simulink model "AXIS_To_Stream"  (R2018b)
settings: Solver=VariableStepAuto  StartTime=0.0  StopTime=131000*10*10e-9  RelTol=1e-3
libraries: xbsIndex_r4 x29, hdlsllib x1, simulink_extras x1
settings Model: Creator=marsiau  LastModifiedBy=marsiau

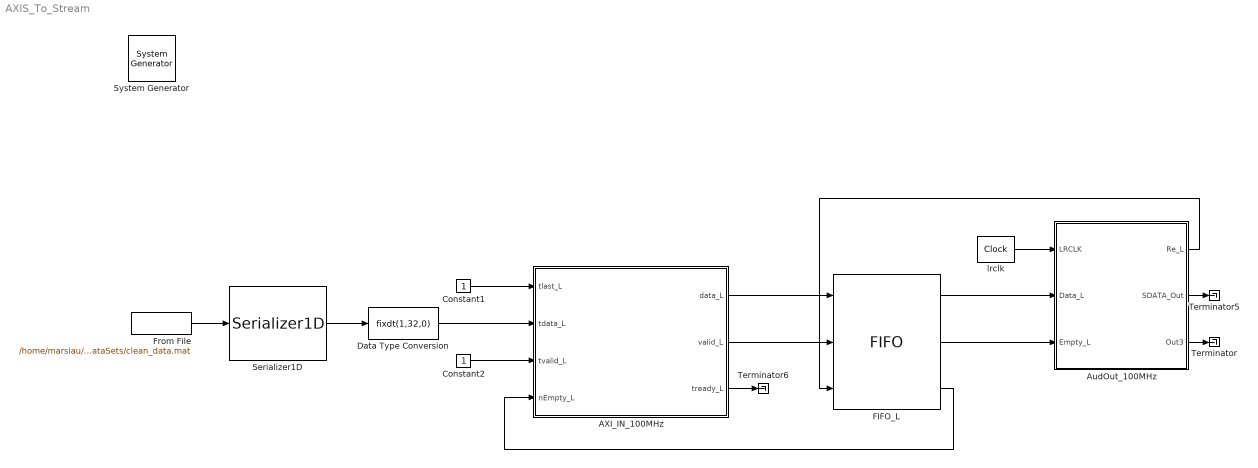
== system AXIS_To_Stream ==
  " System Generator" : xbsIndex_r4/ System Generator  Tag=genX  xilinxfamily=zynq  part=xc7z020  speed=-1  package=clg400  synthesis_tool=Vivado  clock_wrapper=Clock Enables  directory=./netlist  proj_type=Vivado  Synth_file=Vivado Synthesis Defaults  Impl_file=Vivado Implementation Defaults  testbench=off  simulink_period=1  sysclk_period=10  dcm_input_clock_period=10  incr_netlist=off  trim_vbits=Everywhere in SubSystem  dbl_ovrd=According to Block Masks  core_generation=According to Block Masks  run_coregen=off  deprecated_control=off  eval_field=0  block_type=sysgen
  AXI_IN_100MHz : Subsystem
  AudOut_100MHz : Subsystem
  Constant1 : Constant  OutDataTypeStr=boolean  SampleTime=10e-9
  Constant2 : Constant  OutDataTypeStr=boolean  SampleTime=10e-9
  Data Type Conversion : DataTypeConversion  OutDataTypeStr=fixdt(1,32,0)  SaturateOnIntegerOverflow=on  LockScale=on
  FIFO_L : xbsIndex_r4/FIFO  mem_type=Block RAM  performance_options=Standard_FIFO  embedded_registers=off  depth=16K  percent_nbits=1  rst=off  rst_latency=1  en=off  use_dcount=off  use_percent_full_port=off  use_almost_empty=off  almost_empty_thresh=2  use_almost_full=off  use_rd_rst_busy=off  use_wr_rst_busy=off  almost_full_thresh=14  explicit_period=off  dbl_ovrd=off  block_type=fifo
  From File : FromFile  FileName=/home/marsiau/Projects/PYNQ-RTL-SDR/IP/DataSets/clean_data.mat
  Serializer1D : hdlsllib/HDL Operations/Serializer1D  Ratio=131000  IdleCycles=0  validIn=off  startOut=off  validOut=off  inputDataDimensions=-1  inputSampleTime=-1  inputSignalType=auto
      settings: SourceProductName=HDL Coder  SourceProductBaseCode=HD
  Terminator : Terminator
  Terminator5 : Terminator
  Terminator6 : Terminator
  lrclk : simulink_extras/Flip Flops/Clock  period=20.48e-6
  wires:
  FIFO_L/2 -> AudOut_100MHz/3(Empty_L)
  AXI_IN_100MHz/3(tready_L) -> Terminator6/1
  FIFO_L/1 -> AudOut_100MHz/2(Data_L)
  lrclk/1 -> AudOut_100MHz/1(LRCLK)
  AXI_IN_100MHz/2(valid_L) -> FIFO_L/2
  From File/1 -> Serializer1D/1
  AudOut_100MHz/2(SDATA_Out) -> Terminator5/1
  AXI_IN_100MHz/1(data_L) -> FIFO_L/1
  Data Type Conversion/1 -> AXI_IN_100MHz/2(tdata_L)
  FIFO_L/3 -> AXI_IN_100MHz/4(nEmpty_L)
  Constant1/1 -> AXI_IN_100MHz/1(tlast_L)
  AudOut_100MHz/3(Out3) -> Terminator/1
  AudOut_100MHz/1(Re_L) -> FIFO_L/3
  Serializer1D/1 -> Data Type Conversion/1
  Constant2/1 -> AXI_IN_100MHz/3(tvalid_L)

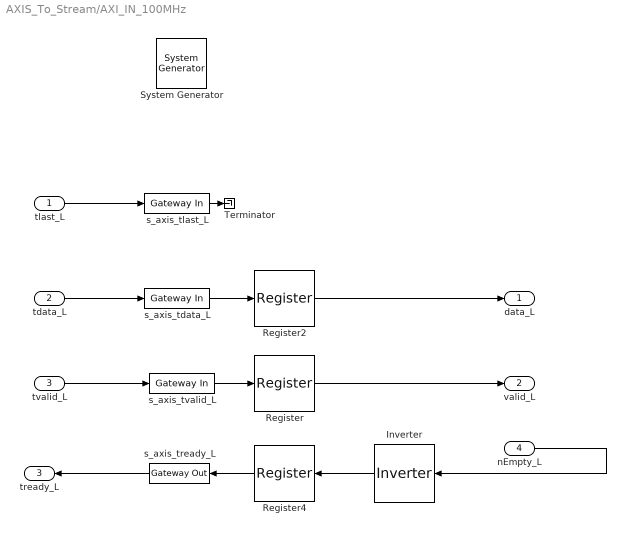
== system AXIS_To_Stream/AXI_IN_100MHz ==
  tlast_L : Inport
  tdata_L : Inport  Port=2
  tvalid_L : Inport  Port=3
  nEmpty_L : Inport  Port=4
  " System Generator" : xbsIndex_r4/ System Generator  Tag=genX  xilinxfamily=zynq  part=xc7z020  speed=-1  package=clg400  synthesis_tool=Vivado  clock_wrapper=Clock Enables  directory=./netlist  proj_type=Vivado  Synth_file=Vivado Synthesis Defaults  Impl_file=Vivado Implementation Defaults  testbench=off  simulink_period=10e-9  sysclk_period=10  dcm_input_clock_period=10  incr_netlist=off  trim_vbits=Everywhere in SubSystem  dbl_ovrd=According to Block Masks  core_generation=According to Block Masks  run_coregen=off  deprecated_control=off  eval_field=0  block_type=sysgen
  Inverter : xbsIndex_r4/Inverter  en=off  latency=0  dbl_ovrd=off  block_type=inv
  Register : xbsIndex_r4/Register  init=0  rst=off  en=off  dbl_ovrd=off  block_type=register
  Register2 : xbsIndex_r4/Register  init=0  rst=off  en=off  dbl_ovrd=off  block_type=register
  Register4 : xbsIndex_r4/Register  init=0  rst=off  en=off  dbl_ovrd=off  block_type=register
  Terminator : Terminator
  s_axis_tdata_L : xbsIndex_r4/Gateway In  gui_display_data_type=Fixed-point  arith_type=Unsigned  n_bits=32  bin_pt=0  preci_type=Single  exp_width=8  frac_width=24  rows=1  columns=1  quantization="Round  (unbiased: +/- Inf)"  overflow=Saturate  period=10e-9  UseAsADC=off  ADCChannel='1'  interface=None  automatic_assignment=on  address_offset=hex2dec('00')  intf_name=''  intf_description=''  default_value=0  timing_constraint=None  locs_specified=off  LOCs={}  io_standard={}  inherit_from_input=off  hdl_port=on  dbl_ovrd=off  block_type=gatewayin
  s_axis_tlast_L : xbsIndex_r4/Gateway In  gui_display_data_type=Boolean  arith_type=Boolean  n_bits=16  bin_pt=14  preci_type=Single  exp_width=8  frac_width=24  rows=1  columns=1  quantization="Round  (unbiased: +/- Inf)"  overflow=Saturate  period=10e-9  UseAsADC=off  ADCChannel='1'  interface=None  automatic_assignment=on  address_offset=hex2dec('00')  intf_name=''  intf_description=''  default_value=0  timing_constraint=None  locs_specified=off  LOCs={}  io_standard={}  inherit_from_input=off  hdl_port=on  dbl_ovrd=off  block_type=gatewayin
  s_axis_tready_L : xbsIndex_r4/Gateway Out  inherit_from_input=off  hdl_port=on  rows=1  columns=1  UseAsDAC=off  DACChannel='1'  interface=None  automatic_assignment=on  address_offset=hex2dec('00')  intf_name=''  intf_description=''  timing_constraint=None  locs_specified=off  LOCs={}  io_standard={}  block_type=gatewayout
  s_axis_tvalid_L : xbsIndex_r4/Gateway In  gui_display_data_type=Boolean  arith_type=Boolean  n_bits=16  bin_pt=14  preci_type=Single  exp_width=8  frac_width=24  rows=1  columns=1  quantization="Round  (unbiased: +/- Inf)"  overflow=Saturate  period=10e-9  UseAsADC=off  ADCChannel='1'  interface=None  automatic_assignment=on  address_offset=hex2dec('00')  intf_name=''  intf_description=''  default_value=0  timing_constraint=None  locs_specified=off  LOCs={}  io_standard={}  inherit_from_input=off  hdl_port=on  dbl_ovrd=off  block_type=gatewayin
  data_L : Outport
  valid_L : Outport  Port=2
  tready_L : Outport  Port=3
  wires:
  s_axis_tvalid_L/1 -> Register/1
  s_axis_tdata_L/1 -> Register2/1
  s_axis_tlast_L/1 -> Terminator/1
  Inverter/1 -> Register4/1
  s_axis_tready_L/1 -> tready_L/1
  tlast_L/1 -> s_axis_tlast_L/1
  tvalid_L/1 -> s_axis_tvalid_L/1
  tdata_L/1 -> s_axis_tdata_L/1
  nEmpty_L/1 -> Inverter/1
  Register/1 -> valid_L/1
  Register4/1 -> s_axis_tready_L/1
  Register2/1 -> data_L/1

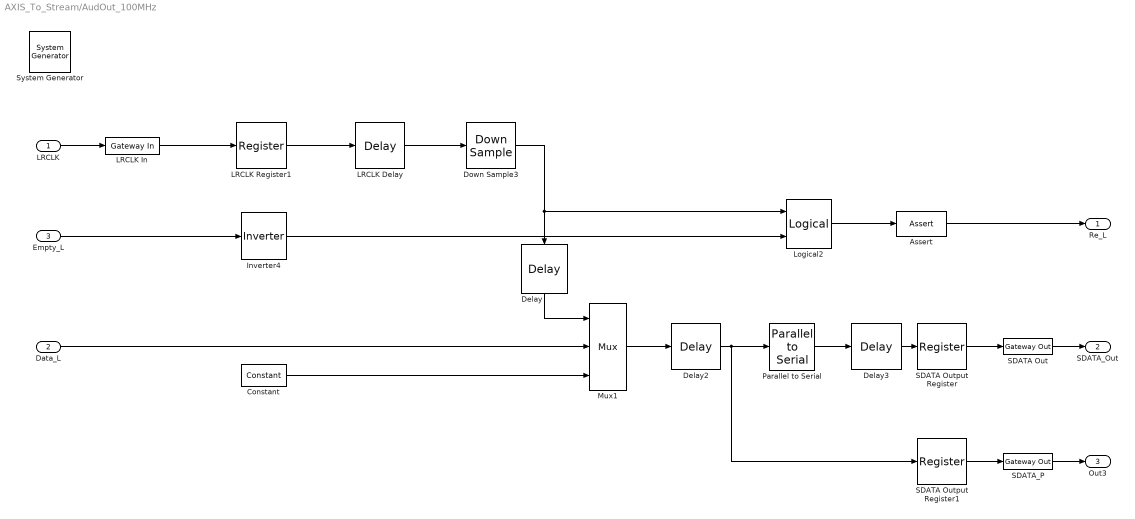
== system AXIS_To_Stream/AudOut_100MHz ==
  LRCLK : Inport
  Data_L : Inport  Port=2
  Empty_L : Inport  Port=3
  " System Generator" : xbsIndex_r4/ System Generator  Tag=genX  xilinxfamily=zynq  part=xc7z020  speed=-1  package=clg400  synthesis_tool=Vivado  clock_wrapper=Clock Enables  directory=./netlist  proj_type=Vivado  Synth_file=Vivado Synthesis Defaults  Impl_file=Vivado Implementation Defaults  testbench=off  simulink_period=10e-9  sysclk_period=10  dcm_input_clock_period=10  incr_netlist=off  trim_vbits=Everywhere in SubSystem  dbl_ovrd=According to Block Masks  core_generation=According to Block Masks  run_coregen=off  deprecated_control=off  eval_field=0  block_type=sysgen
  Assert : xbsIndex_r4/Assert  assert_type=off  type_source=Explicitly  gui_display_data_type=Fixed-point  arith_type="Signed  (2's comp)"  n_bits=16  bin_pt=14  preci_type=Single  exp_width=8  frac_width=24  assert_rate=on  rate_source=Explicitly  period=10.24e-6  output_port=on  block_type=assert
  Constant : xbsIndex_r4/Constant  const=0  gui_display_data_type=Fixed-point  arith_type=Unsigned  n_bits=32  bin_pt=0  preci_type=Single  exp_width=8  frac_width=24  explicit_period=on  period=10.24e-6  equ=P=C  opselect=C  inp2=PCIN>>17  opr=+  inp1=P  carry=CIN  dbl_ovrd=off  block_type=constant
  Delay : xbsIndex_r4/Delay  rst=off  infoeditControl=Selection of Reset will increase slice count due to use of real FFs and instead of SRLs  en=off  latency=1  reg_retiming=off  dbl_ovrd=off  block_type=delay
  Delay2 : xbsIndex_r4/Delay  rst=off  infoeditControl=Selection of Reset will increase slice count due to use of real FFs and instead of SRLs  en=off  latency=1  reg_retiming=off  dbl_ovrd=off  block_type=delay
  Delay3 : xbsIndex_r4/Delay  rst=off  infoeditControl=Selection of Reset will increase slice count due to use of real FFs and instead of SRLs  en=off  latency=32  reg_retiming=off  dbl_ovrd=off  block_type=delay
  Down Sample3 : xbsIndex_r4/Down Sample  sample_ratio=1024  sample_phase=First Value of Frame  en=off  rst=off  latency=0  dbl_ovrd=off  block_type=dsamp
  Inverter4 : xbsIndex_r4/Inverter  en=off  latency=1  dbl_ovrd=off  block_type=inv
  LRCLK Delay : xbsIndex_r4/Delay  rst=off  infoeditControl=Selection of Reset will increase slice count due to use of real FFs and instead of SRLs  en=off  latency=31  reg_retiming=off  dbl_ovrd=off  block_type=delay
  LRCLK In : xbsIndex_r4/Gateway In  gui_display_data_type=Boolean  arith_type=Boolean  n_bits=1  bin_pt=0  preci_type=Single  exp_width=8  frac_width=24  rows=1  columns=1  quantization=Truncate  overflow=Saturate  period=10e-9  UseAsADC=off  ADCChannel='1'  interface=None  automatic_assignment=off  address_offset=hex2dec('04')  intf_name=''  intf_description=''  default_value=0  timing_constraint=None  locs_specified=off  LOCs={}  io_standard={}  inherit_from_input=off  hdl_port=on  dbl_ovrd=off  block_type=gatewayin
  LRCLK Register1 : xbsIndex_r4/Register  init=0  rst=off  en=off  dbl_ovrd=off  block_type=register
  Logical2 : xbsIndex_r4/Logical  logical_function=AND  inputs=2  en=off  latency=1  precision=Full  arith_type=Unsigned  n_bits=16  bin_pt=0  align_bp=on  dbl_ovrd=off  block_type=logical
  Mux1 : xbsIndex_r4/Mux  inputs=2  en=off  latency=1  precision=Full  arith_type=Unsigned  n_bits=16  bin_pt=14  quantization=Truncate  overflow=Wrap  dbl_ovrd=off  block_type=mux
  Parallel to Serial : xbsIndex_r4/Parallel to Serial  output_order=Most Significant Word First  arith_type=Unsigned  output_bits=1  bin_pt=0  rst=off  en=off  latency=0  dbl_ovrd=off  block_type=p2s
      settings: infoedit=Each sample presented at the input becomes several samples presented serially at the output.
  SDATA Out : xbsIndex_r4/Gateway Out  inherit_from_input=on  hdl_port=on  rows=1  columns=1  UseAsDAC=off  DACChannel='1'  interface=None  automatic_assignment=on  address_offset=hex2dec('00')  intf_name=''  intf_description=''  timing_constraint=None  locs_specified=off  LOCs={}  io_standard={}  block_type=gatewayout
  SDATA Output Register : xbsIndex_r4/Register  init=0  rst=off  en=off  dbl_ovrd=off  block_type=register
  SDATA Output Register1 : xbsIndex_r4/Register  init=0  rst=off  en=off  dbl_ovrd=off  block_type=register
  SDATA_P : xbsIndex_r4/Gateway Out  inherit_from_input=on  hdl_port=on  rows=1  columns=1  UseAsDAC=off  DACChannel='1'  interface=None  automatic_assignment=on  address_offset=hex2dec('00')  intf_name=''  intf_description=''  timing_constraint=None  locs_specified=off  LOCs={}  io_standard={}  block_type=gatewayout
  Re_L : Outport
  SDATA_Out : Outport  Port=2
  Out3 : Outport  Port=3
  wires:
  SDATA Output Register/1 -> SDATA Out/1
  Mux1/1 -> Delay2/1
  LRCLK In/1 -> LRCLK Register1/1
  LRCLK Register1/1 -> LRCLK Delay/1
  SDATA Out/1 -> SDATA_Out/1
  Parallel to Serial/1 -> Delay3/1
  LRCLK/1 -> LRCLK In/1
  Empty_L/1 -> Inverter4/1
  LRCLK Delay/1 -> Down Sample3/1
  Down Sample3/1 -> Delay/1, Logical2/1
  Logical2/1 -> Assert/1
  Inverter4/1 -> Logical2/2
  Data_L/1 -> Mux1/2
  Assert/1 -> Re_L/1
  Constant/1 -> Mux1/3
  Delay/1 -> Mux1/1
  SDATA Output Register1/1 -> SDATA_P/1
  Delay2/1 -> SDATA Output Register1/1, Parallel to Serial/1
  SDATA_P/1 -> Out3/1
  Delay3/1 -> SDATA Output Register/1
